simulink model "M_3DoF_Continuous_PID_with_Aero_4"  (R2020b)
settings: Solver=VariableStepAuto  StartTime=0.0  StopTime=3.5  RelTol=1e-3
undefined symbols (not defined in the file or in its folder): air_density, Cd, cg2cp, Cl, ref_area
libraries: simulink_extras x3, shared3dof x1, pid_lib x1
settings Model: Creator=raghavendrans  LastModifiedBy=raghavendrans

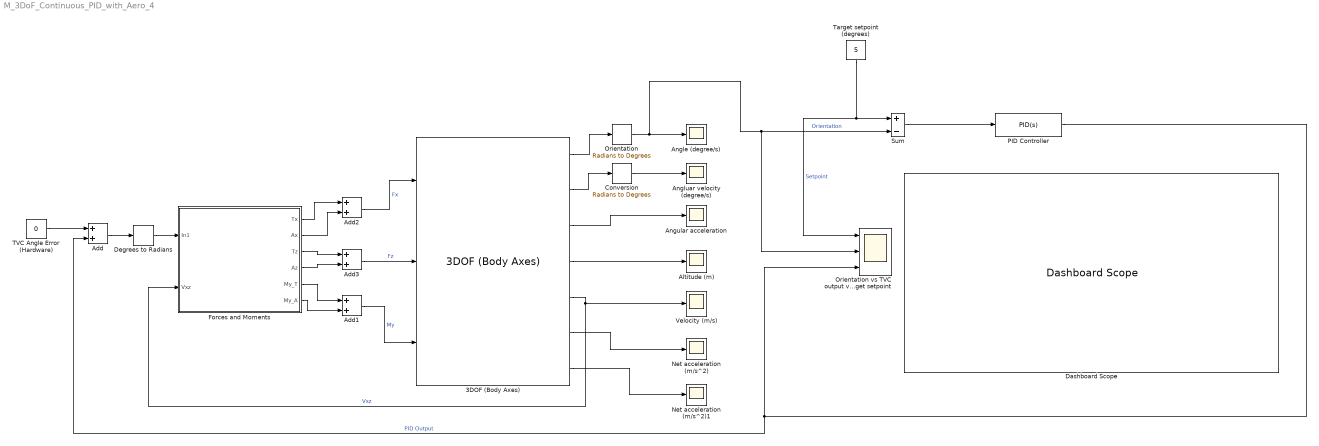
== system M_3DoF_Continuous_PID_with_Aero_4 ==
  3DOF (Body Axes) : shared3dof/3DOF (Body Axes)  units=Metric (MKS)  mtype=Fixed  v_ini=0  theta_ini=0  alpha_ini=0  pos_ini=[0 0]  q_ini=0  mass=mass  mass_e=0.5  mass_f=3.0  Iyy=0.048  Iyy_e=0.5  Iyy_f=3.0  g_in=Internal  g=-9.81  vre_flag=on  abi_flag=on  aMode=0  vel_statename=''  theta_statename=''  pos_statename=''  q_statename=''  mass_statename=''
      settings: SourceProductBaseCode=AE,PW,MT,UV,VE,VP
  Add{,1..3} (4 alike) : Sum
  Altitude (m) : Scope
  Angle (degree/s) : Scope
  Angluar velocity (degree/s) : Scope
  Angular acceleration : Scope
  Conversion : simulink_extras/Transformations/Radians to Degrees
  Dashboard Scope : DashboardScope
  Degrees to Radians : simulink_extras/Transformations/Degrees to Radians
  Forces and Moments : Subsystem
  Net acceleration (m/s^2) : Scope
  Net acceleration (m/s^2)1 : Scope
  Orientation : simulink_extras/Transformations/Radians to Degrees
  Orientation vs TVC output vs Target setpoint : Scope  NumInputPorts=3
  PID Controller : pid_lib/PID Controller  Controller=PID  Form=Parallel  TimeDomain=Continuous-time  UseExternalTs=off  SampleTime=-1  IntegratorMethod=Forward Euler  FilterMethod=Forward Euler  ControllerParametersSource=internal  P=1  I=3  D=0.08  UseFilter=on  N=100  TunerSelectOption=Transfer Function Based (PID Tuner App)  InitialConditionSource=internal  InitialConditionForIntegrator=0  InitialConditionForFilter=0  DifferentiatorICPrevScaledInput=0  ExternalReset=none  TrackingMode=off  Kt=1  LimitOutput=on  SatLimitsSource=internal  UpperSaturationLimit=5  LowerSaturationLimit=-5  LinearizeAsGain=on  AntiWindupMode=none  Kb=1  POutMin=[]  POutMax=[]  IOutMin=[]  IOutMax=[]  DOutMin=[]  DOutMax=[]  NOutMin=[]  NOutMax=[]  SumOutMin=[]  SumOutMax=[]  SaturationOutMin=[]  SaturationOutMax=[]  PParamMin=[]  PParamMax=[]  IParamMin=[]  IParamMax=[]  DParamMin=[]  DParamMax=[]  NParamMin=[]  NParamMax=[]  KbParamMin=[]  KbParamMax=[]  KtParamMin=[]  KtParamMax=[]  KbOutMin=[]  KbOutMax=[]  KtOutMin=[]  KtOutMax=[]  IntegratorOutMin=[]  IntegratorOutMax=[]  FilterOutMin=[]  FilterOutMax=[]  SumI1OutMin=[]  SumI1OutMax=[]  SumI2OutMin=[]  SumI2OutMax=[]  SumI3OutMin=[]  SumI3OutMax=[]  SumI4OutMin=[]  SumI4OutMax=[]  SumDOutMin=[]  SumDOutMax=[]  DifferentiatorOutMin=[]  DifferentiatorOutMax=[]  FilterDiffOutCoefMin=[]  FilterDiffOutCoefMax=[]  ReciprocalOutMin=[]  ReciprocalOutMax=[]  SumDenOutMin=[]  SumDenOutMax=[]  SumNumOutMin=[]  SumNumOutMax=[]  DivideOutMin=[]  DivideOutMax=[]  UdiffTsProdOutMin=[]  UdiffTsProdOutMax=[]  NTsProdOutMin=[]  NTsProdOutMax=[]  UintegralTsProdOutMin=[]  UintegralTsProdOutMax=[]  UngainTsProdOutMin=[]  UngainTsProdOutMax=[]  IntegratorContinuousStateAttributes=''  IntegratorStateMustResolveToSignalObject=off  IntegratorRTWStateStorageClass=Auto  FilterContinuousStateAttributes=''  FilterStateMustResolveToSignalObject=off  FilterRTWStateStorageClass=Auto  ParallelPVariant=InternalParameters  IdealPVariant=Disabled  IVariant=InternalParameters  DVariant=InternalParameters  IntegratorVariant=Continuous  SatVariant=Enabled  AWVariant=Passthrough  PCopyVariant=Disabled  TRVariant=Disabled  FdbkBlocksVariant=Forward  IdealPFdbkVariant=Disabled  SatFdbkVariant=Disabled  DerivativeFilterVariant=ContFilter  NVariant=InternalParameters  NCopyVariant=Disabled  FilterICVariant=InternalICsFilter  IntegratorICVariant=InternalICs  ExternalResetVariant=Disabled  TRSumVariant=Passthrough  SumFdbkVariant=Disabled  SumVariant=Sum_PID  TsampFilterVariant=InternalTs  TsampNgainVariant=Passthrough  TsampIntegralVariant=Passthrough  ExternalSaturationOutDataTypeStr=Inherit: Same as second input
  Sum : Sum  Inputs=+-
  TVC Angle Error (Hardware) : Constant  Value=0
  Target setpoint (degrees) : Constant  Value=5
  Velocity (m/s) : Scope
  wires:
  Add/1 -> Degrees to Radians/1
  TVC Angle Error (Hardware)/1 -> Add/1
  3DOF (Body Axes)/1 -> Orientation/1
  3DOF (Body Axes)/2 -> Conversion/1
  3DOF (Body Axes)/5 -> Forces and Moments/2(Vxz), Velocity (m/s)/1  "Vxz"
  3DOF (Body Axes)/3 -> Angular acceleration/1
  3DOF (Body Axes)/4 -> Altitude (m)/1
  3DOF (Body Axes)/6 -> Net acceleration (m/s^2)/1
  Conversion/1 -> Angluar velocity (degree/s)/1
  Target setpoint (degrees)/1 -> Orientation vs TVC output vs Target setpoint/1, Sum/1  "Setpoint"
  Orientation/1 -> Orientation vs TVC output vs Target setpoint/2, Sum/2, Angle (degree/s)/1  "Orientation"
  PID Controller/1 -> Orientation vs TVC output vs Target setpoint/3, Add/2  "PID Output"
  Sum/1 -> PID Controller/1
  Add1/1 -> 3DOF (Body Axes)/3  "My"
  3DOF (Body Axes)/7 -> Net acceleration (m/s^2)1/1
  Degrees to Radians/1 -> Forces and Moments/1(In1)
  Forces and Moments/1(Tx) -> Add2/1
  Forces and Moments/2(Ax) -> Add2/2
  Forces and Moments/3(Tz) -> Add3/1
  Forces and Moments/4(Az) -> Add3/2
  Forces and Moments/5(My_T) -> Add1/1
  Forces and Moments/6(My_A) -> Add1/2
  Add3/1 -> 3DOF (Body Axes)/2  "Fz"
  Add2/1 -> 3DOF (Body Axes)/1  "Fx"

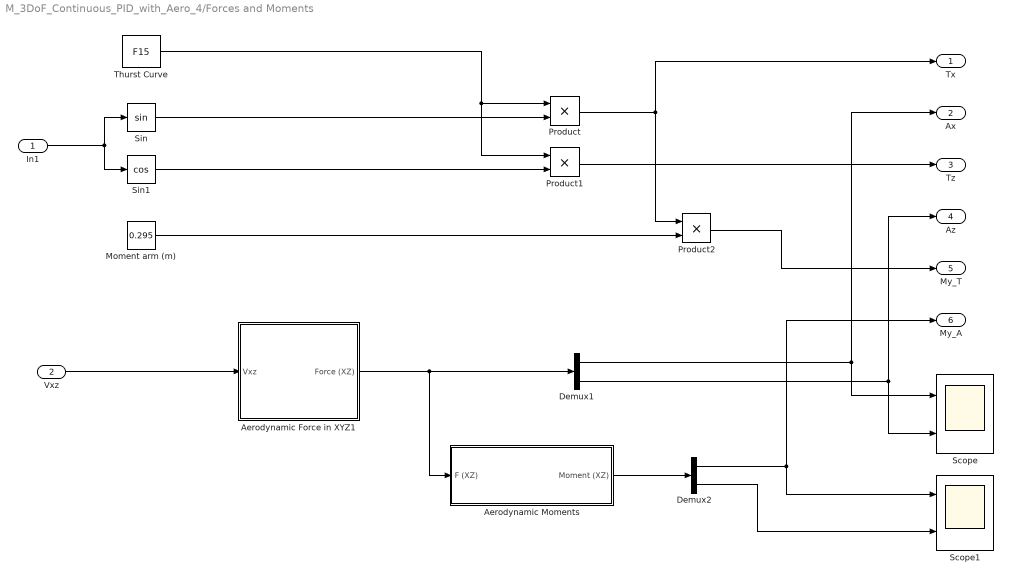
== system M_3DoF_Continuous_PID_with_Aero_4/Forces and Moments ==
  In1 : Inport
  Vxz : Inport  Port=2
  Aerodynamic Force in XYZ1 : Subsystem
  Aerodynamic Moments : Subsystem
  Demux1 : Demux  Outputs=2
  Demux2 : Demux  Outputs=2
  Moment arm (m) : Constant  Value=0.295
  Product : Product
  Product1 : Product
  Product2 : Product
  Scope : Scope  NumInputPorts=2
  Scope1 : Scope  NumInputPorts=2
  Sin : Trigonometry
  Sin1 : Trigonometry  Operator=cos
  Thurst Curve : FromWorkspace  VariableName=F15
  Tx : Outport
  Ax : Outport  Port=2
  Tz : Outport  Port=3
  Az : Outport  Port=4
  My_T : Outport  Port=5
  My_A : Outport  Port=6
  wires:
  Vxz/1 -> Aerodynamic Force in XYZ1/1(Vxz)
  Product2/1 -> My_T/1
  Demux2/2 -> Scope1/2
  Aerodynamic Force in XYZ1/1(Force (XZ)) -> Demux1/1, Aerodynamic Moments/1(F (XZ))
  Demux2/1 -> Scope1/1, My_A/1
  Aerodynamic Moments/1(Moment (XZ)) -> Demux2/1
  Product/1 -> Product2/1, Tx/1
  Product1/1 -> Tz/1
  Demux1/1 -> Scope/1, Ax/1
  Demux1/2 -> Scope/2, Az/1
  Sin1/1 -> Product1/2
  Moment arm (m)/1 -> Product2/2
  Sin/1 -> Product/2
  In1/1 -> Sin1/1, Sin/1
  Thurst Curve/1 -> Product1/1, Product/1

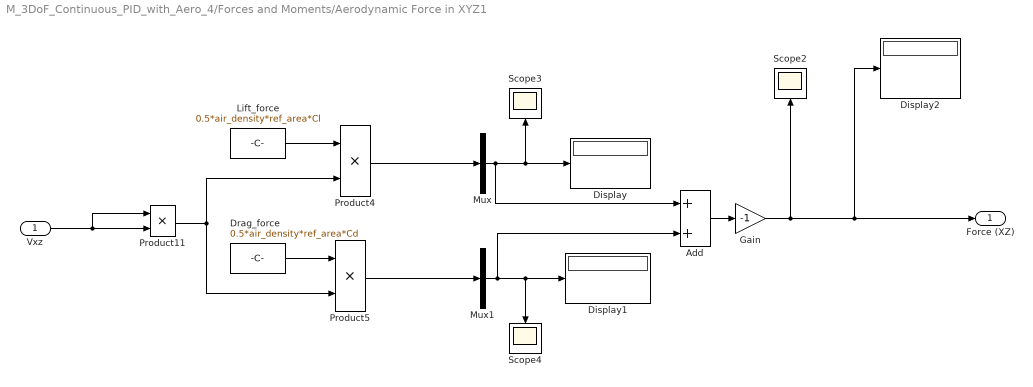
== system M_3DoF_Continuous_PID_with_Aero_4/Forces and Moments/Aerodynamic Force in XYZ1 ==
  Vxz : Inport
  Add : Sum
  Display : Display
  Display1 : Display
  Display2 : Display
  Drag_force : Constant  Value=0.5*air_density*ref_area*Cd
  Gain : Gain  Gain=-1
  Lift_force : Constant  Value=0.5*air_density*ref_area*Cl
  Mux : Mux  Inputs=1
  Mux1 : Mux  Inputs=1
  Product11 : Product
  Product4 : Product
  Product5 : Product
  Scope2 : Scope
  Scope3 : Scope
  Scope4 : Scope
  Force (XZ) : Outport
  wires:
  Lift_force/1 -> Product4/1
  Vxz/1 -> Product11/1, Product11/2
  Drag_force/1 -> Product5/1
  Product11/1 -> Product4/2, Product5/2
  Mux/1 -> Add/1, Scope3/1, Display/1
  Product4/1 -> Mux/1
  Product5/1 -> Mux1/1
  Mux1/1 -> Add/2, Scope4/1, Display1/1
  Add/1 -> Gain/1
  Gain/1 -> Scope2/1, Display2/1, Force (XZ)/1

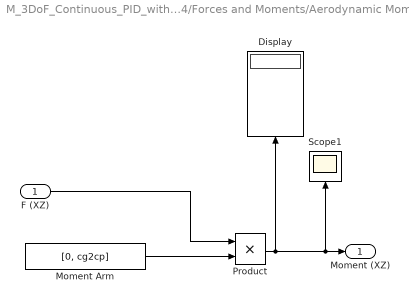
== system M_3DoF_Continuous_PID_with_Aero_4/Forces and Moments/Aerodynamic Moments ==
  F (XZ) : Inport
  Display : Display
  Moment Arm : Constant  Value=[0, cg2cp]
  Product : Product
  Scope1 : Scope
  Moment (XZ) : Outport
  wires:
  Product/1 -> Moment (XZ)/1, Scope1/1, Display/1
  Moment Arm/1 -> Product/2
  F (XZ)/1 -> Product/1
